simulink model "prova"  (R2023a)
settings: Solver=VariableStepAuto  StartTime=0.0  StopTime=10  RelTol=1e-3
values from neighbouring files (symbols this model uses):
  A = vpa(subs(jacobian(fx + gx*u, x), u, u_e),2)    [LinSym.m]    (also in PlotPendubot.m = double(vpa(subs(jacobian(fx + gx*u, x), [x; u], [x_e; u_e]),; sim_ode45.m = double(vpa(subs(jacobian(fx + gx*u, x), [x; u], [x_e; u_e]),)
  B = vpa(subs(jacobian(fx + gx*u, u), u, u_e),2)    [LinSym.m]    (also in PlotPendubot.m = double(vpa(subs(jacobian(fx + gx*u, u), x, x_e), 3)); sim_ode45.m = double(vpa(subs(jacobian(fx + gx*u, u), x, x_e), 3)))
  C = eye(n)    [PlotPendubot.m]    (also in sim_ode45.m)
  D = zeros(n,1)    [PlotPendubot.m]    (also in sim_ode45.m)
  u_e = vpa(solve(subs(x_dot, x, x_e), u),5)    [LinSym.m]    (also in PlotPendubot.m = double(vpa(solve(subs(eqns, x, x_e ), u), 5)); sim_ode45.m = double(vpa(solve(subs(eqns, x, x_e ), u), 5)))
  x_e = [4*pi/3; pi; 0; 0]    [PlotPendubot.m]    (also in SolveSyms.m = [pi; pi; 0; 0]; sim_ode45.m = [4/3*pi; pi; 0; 0])
  x_ini = [pi; pi; 0; 0]    [PlotPendubot.m]    (also in SolveSyms.m = [pi/24; 0; 0; 0]; sim_ode45.m)
settings Model: Creator=Pc Lorenzo  LastModifiedBy=Pc Lorenzo

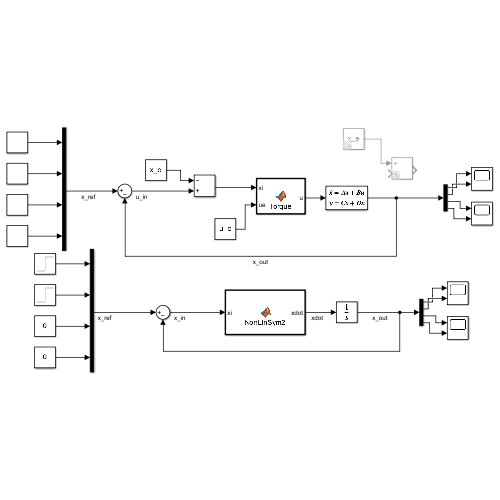
[thumbnail: Simulink's stored preview of the top-level diagram]
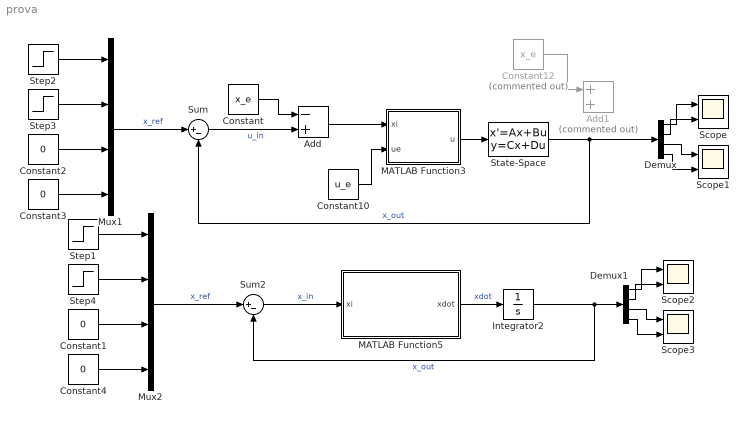
== system prova ==
  Add : Sum  Inputs=-+
  Add1 : Sum  Commented=on
  Constant : Constant  Value=x_e
  Constant{1..4} (4 alike) : Constant  Value=0
  Constant10 : Constant  Value=u_e
  Constant12 : Constant  Commented=on  Value=x_e
  Demux : Demux
  Demux1 : Demux
  Integrator2 : Integrator  InitialCondition=x_ini
  MATLAB Function3 : MATLAB Function  TreatAsAtomicUnit=on
  MATLAB Function5 : MATLAB Function  TreatAsAtomicUnit=on
  Mux1 : Mux
  Mux2 : Mux
  Scope{,1..3} (4 alike) : Scope  NumInputPorts=2
  State-Space : StateSpace  A=A  B=B  C=C  D=D  InitialCondition=x_ini
  Step1 : Step  Before=pi  After=4/3 * pi  SampleTime=0
  Step2 : Step  Before=pi  After=4/3 * pi  SampleTime=0
  Step3 : Step  Before=pi  After=pi  SampleTime=0
  Step4 : Step  Before=pi  After=pi  SampleTime=0
  Sum : Sum  Inputs=|+-
  Sum2 : Sum  Inputs=|+-
  wires:
  Mux1/1 -> Sum/1  "x_ref"
  Sum/1 -> Add/2  "u_in"
  State-Space/1 -> Demux/1, Sum/2  "x_out"
  MATLAB Function3/1(u) -> State-Space/1
  Constant10/1 -> MATLAB Function3/2(ue)
  MATLAB Function5/1(xdot) -> Integrator2/1  "xdot"
  Mux2/1 -> Sum2/1  "x_ref"
  Constant/1 -> Add/1
  Add/1 -> MATLAB Function3/1(xi)
  Sum2/1 -> MATLAB Function5/1(xi)  "x_in"
  Demux/1 -> Scope/1
  Demux/2 -> Scope/2
  Demux/3 -> Scope1/1
  Demux/4 -> Scope1/2
  Demux1/2 -> Scope2/2
  Demux1/4 -> Scope3/2
  Demux1/1 -> Scope2/1
  Demux1/3 -> Scope3/1
  Constant12/1 -> Add1/1
  Constant3/1 -> Mux1/4
  Constant2/1 -> Mux1/3
  Step2/1 -> Mux1/1
  Step3/1 -> Mux1/2
  Constant4/1 -> Mux2/4
  Constant1/1 -> Mux2/3
  Step1/1 -> Mux2/1
  Step4/1 -> Mux2/2
  Integrator2/1 -> Sum2/2, Demux1/1  "x_out"

== matlab function prova/MATLAB Function3 ==
  data: xi input; u output; ue input
function u = Torque(xi, ue)
x=[xi(1); xi(3); xi(2); xi(4)]; % state vector alpha1, alpha2, dalpha1/dt, dalpha2/dt

p1=0.0148;%kg m^2
p2=0.0051;
p3=0.0046;
p4=0.1003;%kg m
p5=0.0303;
g=9.81;

k = 3.9621/8;%V (Nm)^â?»1

%M(alpha)
m11 = p1 + p2 + 2*p3*cos(x(2)-x(1));  m12 = p2 + p3*cos(x(2)-x(1));
m21 = p2 + p3*cos(x(2)-x(1));         m22 = p2;
M=[m11 m12; m21 m22];

%Vm(alpha, dalpha/dt)*dalpha/dt
Vmda = p3*sin(x(2)-x(1))*[-x(4)*x(3) + x(3)^2 - x(4)^2 ; x(3)^2];

%G(alpha)
G = [p4*g*sin(x(1)); p5*g*sin(x(2))];

% Torque
% tau = M*[x(3); x(4)] + Vmda + G;
d2a = 3*x(1)-0.3*x(3);
tau = (m11 - m12*m21/m22)*d2a + (Vmda(1) - m12*Vmda(2)/m22) + G(1) - m12*G(2)/m22;
u = tau/k - ue;
% u = - ue;

== matlab function prova/MATLAB Function5 ==
  data: xdot output; xi input
function xdot =NonLinSym2(xi)

%pendubot's equations
y = zeros(4,1);
x = [xi(1); xi(2); xi(3); xi(4)]; % state vector alpha1, alpha2, dalpha1/dt, dalpha2/dt
% x = xi; % state vector alpha1, alpha2, dalpha1/dt, dalpha2/dt

p1=0.0148;%kg m^2
p2=0.0051;
p3=0.0046;
p4=0.1003;%kg m
p5=0.0303;
g=9.81;

k = 3.9621/8;%V (Nm)^â?»1

%M(alpha)
m11 = p1 + p2 + 2*p3*cos(x(2)-x(1));  m12 = p2 + p3*cos(x(2)-x(1));
m21 = p2 + p3*cos(x(2)-x(1));         m22 = p2;
M=[m11 m12; m21 m22];

%Vm(alpha, dalpha/dt)*dalpha/dt
Vmda = p3*sin(x(2)-x(1))*[-x(4)*x(3) + x(3)^2 - x(4)^2 ; x(3)^2];

%G(alpha)
G = [p4*g*sin(x(1)); p5*g*sin(x(2))];

% fx = [x(3); x(4); M\(-Vm*[x(3); x(4)] - G)];
fx = [x(3); x(4); M\(-Vmda - G)];
gx = [0; 0; M\[k; 0]];

% Torque
% tau = M*[x(3); x(4)] + Vmda + G;

% d2a = 3*x(1)-0.3*x(3);
% tau = (m11 - m12*m21/m22)*d2a + (Vmda(1)-m12*Vmda(2)/m22) + (G(1) - m12*G(2)/m22);
% u = tau/k;

u = 3*x(1)+0.3*x(3);
% u = 0;

% new state vector
xdot = fx + gx.*u;
% y = x;
